simulink model "Marine_LocoMotive_UAV"  (R2018a)
settings: Solver=ode4  StartTime=0.0  StopTime=80  FixedStep=T  RelTol=1e-3
values from neighbouring files (symbols this model uses):
  a_11 = 0.05*m_b    (= 0.625)    [Marine_LocoMotive_UAV.m]
  a_33 = m_b    (= 12.5)    [Marine_LocoMotive_UAV.m]
  A_w = 1*1.5/2    (= 0.75)    [Marine_LocoMotive_UAV.m]
  A_w2 = 1*0.27/2    (= 0.135)    [Marine_LocoMotive_UAV.m]
  Ac = 0.0331    [Marine_LocoMotive_UAV.m]
  alpha_bar = pi/4    (= 0.785398163397)    [Marine_LocoMotive_UAV.m]
  Am = sysd.denominator{1}    [Marine_LocoMotive_UAV.m]
  Am1_LPF = sysd.denominator{1}    [Marine_LocoMotive_UAV.m]
  Am2_LPF = sysd.denominator{1}    [Marine_LocoMotive_UAV.m]
  Am_asw_LPF = sysd.denominator{1}    [Marine_LocoMotive_UAV.m]
  Am_coup_LPF = sysd.denominator{1}    [Marine_LocoMotive_UAV.m]
  Am_rdeL_LPF = sysd.denominator{1}    [Marine_LocoMotive_UAV.m]
  Am_reL_LPF = sysd.denominator{1}    [Marine_LocoMotive_UAV.m]
  Am_rref20_LPF = sysd.denominator{1}    [Marine_LocoMotive_UAV.m]
  Am_rref_LPF = sysd.denominator{1}    [Marine_LocoMotive_UAV.m]
  AmAlpha_LPF = sysd.denominator{1}    [Marine_LocoMotive_UAV.m]
  Amp_sf = 3    [Marine_LocoMotive_UAV.m]
  AmV_LPF = sysd.denominator{1}    [Marine_LocoMotive_UAV.m]
  AmZ_LPF = sysd.denominator{1}    [Marine_LocoMotive_UAV.m]
  b_11 = 0    [Marine_LocoMotive_UAV.m]
  b_33 = 2*m_b*omega_h    (= 27.5578302946)    [Marine_LocoMotive_UAV.m]
  Bm = sysd.numerator{1}    [Marine_LocoMotive_UAV.m]
  Bm1_LPF = sysd.numerator{1}    [Marine_LocoMotive_UAV.m]
  Bm2_LPF = sysd.numerator{1}    [Marine_LocoMotive_UAV.m]
  Bm_asw_LPF = sysd.numerator{1}    [Marine_LocoMotive_UAV.m]
  Bm_coup_LPF = sysd.numerator{1}    [Marine_LocoMotive_UAV.m]
  Bm_rdeL_LPF = sysd.numerator{1}    [Marine_LocoMotive_UAV.m]
  Bm_reL_LPF = sysd.numerator{1}    [Marine_LocoMotive_UAV.m]
  Bm_rref20_LPF = sysd.numerator{1}    [Marine_LocoMotive_UAV.m]
  Bm_rref_LPF = sysd.numerator{1}    [Marine_LocoMotive_UAV.m]
  BmAlpha_LPF = sysd.numerator{1}    [Marine_LocoMotive_UAV.m]
  BmV_LPF = sysd.numerator{1}    [Marine_LocoMotive_UAV.m]
  BmZ_LPF = sysd.numerator{1}    [Marine_LocoMotive_UAV.m]
  C_S = [5;9]*10^-3    [Marine_LocoMotive_UAV.m]
  Cd_u = 0.2    [Marine_LocoMotive_UAV.m]
  D_x = b_11 + D_s(1)    [Marine_LocoMotive_UAV.m]
  D_z = b_33 + D_s(2)    [Marine_LocoMotive_UAV.m]
  dc_M_p = 6.7    [Marine_LocoMotive_UAV.m]
  Delta_h = (A_im/A_b-0.5)*h_b    (= -0.0625)    [Marine_LocoMotive_UAV.m]
  eps_V = 0.1    [Marine_LocoMotive_UAV.m]
  epsilon_1 = 5    [Marine_LocoMotive_UAV.m]
  epsilon_e_u1 = 0.05    [Marine_LocoMotive_UAV.m]
  epsilon_w = 0    [Marine_LocoMotive_UAV.m]
  epsilon_w2 = pi    (= 3.14159265359)    [Marine_LocoMotive_UAV.m]
  g = 9.81    [Marine_LocoMotive_UAV.m]
  gamma_d_p = (2*0.3/0.03*2*0.2*12/4)/10    (= 2.4)    [Marine_LocoMotive_UAV.m]
  H = 10    [Marine_LocoMotive_UAV.m]
  h_b = 0.25    [Marine_LocoMotive_UAV.m]
  J_b = m_b*h_b*l_b/12    (= 0.208333333333)    [Marine_LocoMotive_UAV.m]
  J_u = 0.03    [Marine_LocoMotive_UAV.m]
  K = 40    [Marine_LocoMotive_UAV.m]
  k3 = 24    [Marine_LocoMotive_UAV.m]
  k4 = 0.8    [Marine_LocoMotive_UAV.m]
  k_w = omega_w^2/g    (= 0.123862835563)    [Marine_LocoMotive_UAV.m]
  k_w2 = omega_w2^2/g    (= 0.447144836384)    [Marine_LocoMotive_UAV.m]
  kd_a = 5.6    [Marine_LocoMotive_UAV.m]
  kd_r = 19.5    [Marine_LocoMotive_UAV.m]
  kd_t = 10    [Marine_LocoMotive_UAV.m]
  kd_x = 5    [Marine_LocoMotive_UAV.m]
  kd_z = 2    [Marine_LocoMotive_UAV.m]
  ki_a = 1.6    [Marine_LocoMotive_UAV.m]
  ki_r = 9    [Marine_LocoMotive_UAV.m]
  ki_T = 12    [Marine_LocoMotive_UAV.m]
  ki_x = 1.2    [Marine_LocoMotive_UAV.m]
  ki_z = 1    [Marine_LocoMotive_UAV.m]
  kp_a = 9.6    [Marine_LocoMotive_UAV.m]
  kp_r = 45    [Marine_LocoMotive_UAV.m]
  kp_t = 20    [Marine_LocoMotive_UAV.m]
  kp_T = 25    [Marine_LocoMotive_UAV.m]
  kp_x = 7    [Marine_LocoMotive_UAV.m]
  kp_z = 3    [Marine_LocoMotive_UAV.m]
  L = 0.2    [Marine_LocoMotive_UAV.m]
  l_b = 0.8    [Marine_LocoMotive_UAV.m]
  Lc_0 = 7    [Marine_LocoMotive_UAV.m]
  LIMIT_CMD_PITCH = 45*pi/180    (= 0.785398163397)    [Marine_LocoMotive_UAV.m]
  LIMIT_uCMD_HEIGHT = 3.5*K    (= 140)    [Marine_LocoMotive_UAV.m]
  m_b = rho_w*Vol_b/4    (= 12.5)    [Marine_LocoMotive_UAV.m]
  m_u = 1.8    [Marine_LocoMotive_UAV.m]
  min_sf = 5    [Marine_LocoMotive_UAV.m]
  nu_w = 1.787*10^-6    (= 1.787e-06)    [Marine_LocoMotive_UAV.m]
  omega_w = 2*pi/T_w    (= 1.10231321179)    [Marine_LocoMotive_UAV.m]
  omega_w2 = 2*pi/T_w2    (= 2.09439510239)    [Marine_LocoMotive_UAV.m]
  r_0 = sqrt( (X0_b(1) - X0_u(1))^2 +(X0_b(2) - X0_u(2))^2 )    [Marine_LocoMotive_UAV.m]
  r_bar = Lc_0-0.3    (= 6.7)    [Marine_LocoMotive_UAV.m]
  r_min = (zu_bar-H)-0.2    [Marine_LocoMotive_UAV.m]
  rho_a = 1.225    [Marine_LocoMotive_UAV.m]
  rho_w = 1000    [Marine_LocoMotive_UAV.m]
  T = 1/500    (= 0.002)    [Marine_LocoMotive_UAV.m]
  T_init = 10    [Marine_LocoMotive_UAV.m]
  Theta0 = 0*atan2(V_bar*D_x*cos(alpha_bar_0),V_bar*D_x*sin(alpha_bar_0)+m_u*g*cos(alpha_bar_0))    [Marine_LocoMotive_UAV.m]
  u_s = w_dir*A_w^2*omega_w*k_w*exp(2*k_w*(-Delta_h/2))    [Marine_LocoMotive_UAV.m]
  u_s2 = w_dir2*A_w2^2*omega_w2*k_w2*exp(2*k_w2*(-Delta_h/2))    [Marine_LocoMotive_UAV.m]
  u_t = -1*0.5*1    (= -0.5)    [Marine_LocoMotive_UAV.m]
  u_w = 0*0.2    (= 0)    [Marine_LocoMotive_UAV.m]
  V0_b = [u_t+u_w+u_s+v_x_w, v_z_w]    [Marine_LocoMotive_UAV.m]
  V0_u = [0 0]    [Marine_LocoMotive_UAV.m]
  V_bar = 4    [Marine_LocoMotive_UAV.m]
  Vol_b = A_b*l_b    (= 0.05)    [Marine_LocoMotive_UAV.m]
  w_dir = 1    [Marine_LocoMotive_UAV.m]
  w_dir2 = 1    [Marine_LocoMotive_UAV.m]
  X0_b = [0,H-Delta_h]    [Marine_LocoMotive_UAV.m]
  X0_u = X0_b + [3 3]    [Marine_LocoMotive_UAV.m]
  zu_bar = X0_b(2) + Lc_0*sin(alpha_bar_0)    [Marine_LocoMotive_UAV.m]
undefined symbols (not defined in the file or in its folder): Am_HPF, Am_LPF, Am_LPF2, an1, an1_v, an2, an3, Bm_HPF, Bm_LPF, Bm_LPF2, bn1, bn1_v, bn2, bn3, DiscIntNeverNeededParam, F, Light, magnitude, MIL, OMEGA_FILTER_OUTER, R_b, Tc, Tg, Tn, Ts, Tsc, Tz, X_GPS_offset
libraries: simulink x50, simulink_extras x9, aerolibwind2 x2
(part 6 of 6)

== system Marine_LocoMotive_UAV/UAV controller/u_r_V_Lyapunov buoy velocity/Smooth channel switching1/C1 transition ==
  C1 : Inport
  switch : Inport  Port=2
  C2_0 : Inport  Port=3
  Compare To Constant : simulink/Logic and Bit Operations/Compare To Constant  relop=<  const=0.01  OutDataTypeStr=boolean
  Constant : Constant
  Constant1 : Constant  Value=0.01
  Delay1 : Delay  DelayLength=1
  IC : InitialCondition  Value=0
  Logical Operator : Logic  Operator=NOT  AllPortsSameDT=off  OutDataTypeStr=boolean
  Product : Product
  Subsystem : Subsystem
  Sum : Sum  Inputs=-+|
  Sum1 : Sum  Inputs=++|
  Sum3 : Sum  Inputs=|++
  Switch1 : Switch  Criteria=u2 > Threshold  Threshold=0.5
  Switch2 : Switch  Criteria=u2 > Threshold  Threshold=0.5
  latch : Subsystem  TreatAsAtomicUnit=on
  latch error ON : Scope
  record C2_0 : Subsystem  TreatAsAtomicUnit=on
  smooth transition to C1 : Subsystem  TreatAsAtomicUnit=on
  trigger and reset latch : Subsystem
  C1_trans : Outport
  wires:
  trigger and reset latch/1(Out1) -> latch/Trigger
  Logical Operator/1 -> Product/2
  IC/1 -> latch/1(In1), trigger and reset latch/2(In2)
  switch/1 -> smooth transition to C1/Enable, Subsystem/Enable, trigger and reset latch/1(In1), record C2_0/Trigger, Delay1/1, Logical Operator/1, Switch2/2
  Sum/1 -> smooth transition to C1/1(In1)
  Delay1/1 -> smooth transition to C1/2(reset)
  Compare To Constant/1 -> IC/1
  Subsystem/1(Out1) -> Sum3/1
  Sum3/1 -> Compare To Constant/1
  Product/1 -> Sum3/2  "do not latch C1 is off"
  Constant1/1 -> Product/1
  Constant/1 -> Switch2/3
  Switch2/1 -> latch error ON/1, Switch1/2
  latch/1(Out1) -> Switch2/1
  Switch1/1 -> C1_trans/1  "out"
  C1/1 -> Sum/2, Switch1/1, Subsystem/2(C1)  "C1"
  record C2_0/1(Out1) -> Sum1/1, Sum/1  "C2_0"
  smooth transition to C1/1(Out1) -> Sum1/2
  C2_0/1 -> record C2_0/1(In1)
  Sum1/1 -> Switch1/3, Subsystem/1(addition with C2_0)  "addition with C2_0"

== system Marine_LocoMotive_UAV/UAV controller/u_r_V_Lyapunov buoy velocity/Smooth channel switching1/C2 transition ==
  C2 : Inport
  switch : Inport  Port=2
  C1_0 : Inport  Port=3
  Compare To Constant : simulink/Logic and Bit Operations/Compare To Constant  relop=<  const=0.01  OutDataTypeStr=boolean
  Constant : Constant
  Constant1 : Constant  Value=0.01
  Delay1 : Delay  DelayLength=1
  Logical Operator : Logic  Operator=NOT  AllPortsSameDT=off  OutDataTypeStr=boolean
  Product : Product
  Subsystem : Subsystem
  Sum : Sum  Inputs=-+|
  Sum1 : Sum  Inputs=++|
  Sum3 : Sum  Inputs=|++
  Switch1 : Switch  Criteria=u2 > Threshold  Threshold=0.5
  Switch2 : Switch  Criteria=u2 > Threshold  Threshold=0.5
  latch : Subsystem  TreatAsAtomicUnit=on
  latch error ON : Scope
  record C1_0 : Subsystem  TreatAsAtomicUnit=on
  smooth transition to C1 : Subsystem  TreatAsAtomicUnit=on
  trigger and reset latch : Subsystem
  C2_trans : Outport
  wires:
  trigger and reset latch/1(Out1) -> latch/Trigger
  Compare To Constant/1 -> latch/1(In1), trigger and reset latch/2(In2)
  Subsystem/1(Out1) -> Sum3/1
  Delay1/1 -> smooth transition to C1/2(reset)
  Logical Operator/1 -> Product/2
  Sum3/1 -> Compare To Constant/1
  Constant1/1 -> Product/1
  Product/1 -> Sum3/2
  latch/1(Out1) -> Switch2/1
  Constant/1 -> Switch2/3
  Sum1/1 -> Switch1/3, Subsystem/1(addition with C1_0)  "addition with C1_0"
  C1_0/1 -> record C1_0/1(In1)
  smooth transition to C1/1(Out1) -> Sum1/2
  record C1_0/1(Out1) -> Sum/1, Sum1/1  "C1_0"
  switch/1 -> record C1_0/Trigger, trigger and reset latch/1(trigger), Subsystem/Enable, smooth transition to C1/Enable, Delay1/1, Logical Operator/1, Switch2/2  "trigger"
  Switch2/1 -> latch error ON/1, Switch1/2
  C2/1 -> Switch1/1, Subsystem/2(C2), Sum/2  "C2"
  Switch1/1 -> C2_trans/1  "out"
  Sum/1 -> smooth transition to C1/1(In1)

== system Marine_LocoMotive_UAV/Quadrotor+buoy/3-DOF equations of motion Earth frame/D_123/Water Daming/rotation matrix R body to earth ==
  angle (rad) : Inport
  Gain : Gain  Gain=-1
  Signal Specification1 : SignalSpecification  Dimensions=2
  Signal Specification2 : SignalSpecification  Dimensions=2
  Trigonometric Function1 : Trigonometry  Operator=sincos
  Vector Concatenate1 : Concatenate  Mode=Multidimensional array  ConcatenateDimension=2
  Vector Concatenate2 : Concatenate
  Vector Concatenate3 : Concatenate
  R : Outport
  wires:
  Gain/1 -> Vector Concatenate3/1
  Trigonometric Function1/1 -> Gain/1, Vector Concatenate2/2
  Trigonometric Function1/2 -> Vector Concatenate2/1, Vector Concatenate3/2
  angle (rad)/1 -> Trigonometric Function1/1
  Vector Concatenate3/1 -> Signal Specification2/1
  Vector Concatenate2/1 -> Signal Specification1/1
  Vector Concatenate1/1 -> R/1
  Signal Specification1/1 -> Vector Concatenate1/1
  Signal Specification2/1 -> Vector Concatenate1/2

== system Marine_LocoMotive_UAV/Quadrotor+buoy/3-DOF equations of motion Earth frame/Quadrotor Dynamics Outer-Loop/quadrotor position from relative buoy-UAV position/rotation matrix R  ==
  angle (rad) : Inport
  Gain2 : Gain  Gain=-1
  Gain3 : Gain  Gain=-1
  Signal Specification1 : SignalSpecification  Dimensions=2
  Signal Specification2 : SignalSpecification  Dimensions=2
  Trigonometric Function1 : Trigonometry  Operator=sincos
  Vector Concatenate1 : Concatenate  Mode=Multidimensional array  ConcatenateDimension=2
  Vector Concatenate2 : Concatenate
  Vector Concatenate3 : Concatenate
  R : Outport
  wires:
  Signal Specification2/1 -> Vector Concatenate1/2
  Signal Specification1/1 -> Vector Concatenate1/1
  Vector Concatenate1/1 -> R/1
  Vector Concatenate2/1 -> Signal Specification1/1
  Vector Concatenate3/1 -> Signal Specification2/1
  angle (rad)/1 -> Trigonometric Function1/1
  Trigonometric Function1/1 -> Gain3/1
  Trigonometric Function1/2 -> Vector Concatenate3/2, Gain2/1
  Gain3/1 -> Vector Concatenate2/2, Vector Concatenate3/1
  Gain2/1 -> Vector Concatenate2/1

== system Marine_LocoMotive_UAV/Quadrotor+buoy/3-DOF equations of motion Earth frame/azimuthal dynamics/Coupled System's azimuthal dynamics/azimuth angle dynamics in the coupled system ==
  alpha_ddot : Inport
  alpha init : Inport  Port=2
  alpha dot init : Inport  Port=3
  reset : Inport  Port=4
  Enable : EnablePort
  " alpha" : Scope
  " alpha dot" : Scope
  " alpha dot init" : Scope
  " alpha init" : Scope
  alpha : DiscreteIntegrator  IntegratorMethod=Integration: Backward Euler  ExternalReset=level  InitialConditionSource=external  InitialCondition=alpha_0  SampleTime=-1  ICPrevOutput=DiscIntNeverNeededParam  ICPrevScaledInput=DiscIntNeverNeededParam
  dot(alpha) : DiscreteIntegrator  IntegratorMethod=Integration: Backward Euler  ExternalReset=level  InitialConditionSource=external  SampleTime=-1  ICPrevOutput=DiscIntNeverNeededParam  ICPrevScaledInput=DiscIntNeverNeededParam
  "reset " : Scope
  "alpha " : Outport
  alpha dot : Outport  Port=2
  wires:
  dot(alpha)/1 -> alpha/1, " alpha dot"/1, alpha dot/1
  alpha_ddot/1 -> dot(alpha)/1
  alpha/1 -> "alpha "/1, " alpha"/1
  alpha dot init/1 -> " alpha dot init"/1, dot(alpha)/3
  alpha init/1 -> " alpha init"/1, alpha/3
  reset/1 -> "reset "/1, alpha/2, dot(alpha)/2

== system Marine_LocoMotive_UAV/Quadrotor+buoy/3-DOF equations of motion Earth frame/azimuthal dynamics/Coupled System's azimuthal dynamics/get initial azimuth angle for the coupled dynamics ==
  alpha decoupled : Inport
  alpha dot decoupled : Inport  Port=2
  Trigger : TriggerPort  VariantControl=Variant
  alpha init : Outport
  alpha dot init : Outport  Port=2
  wires:
  alpha decoupled/1 -> alpha init/1
  alpha dot decoupled/1 -> alpha dot init/1

== system Marine_LocoMotive_UAV/Quadrotor+buoy/3-DOF equations of motion Earth frame/azimuthal dynamics/Decoupled System's azimuthal dynamics/magnitude ==
  dX : Inport
  Math Function2 : Math  Operator=square  SaturateOnIntegerOverflow=on
  Sqrt : Sqrt  SaturateOnIntegerOverflow=on
  Sum of Elements : Sum  Inputs=+
  r : Outport
  wires:
  Math Function2/1 -> Sum of Elements/1
  Sum of Elements/1 -> Sqrt/1
  dX/1 -> Math Function2/1
  Sqrt/1 -> r/1

== system Marine_LocoMotive_UAV/Quadrotor+buoy/3-DOF equations of motion Earth frame/azimuthal dynamics/Decoupled System's azimuthal dynamics/rotation matrix R  ==
  angle (rad) : Inport
  Gain : Gain  Gain=-1
  Signal Specification1 : SignalSpecification  Dimensions=2
  Signal Specification2 : SignalSpecification  Dimensions=2
  Trigonometric Function1 : Trigonometry  Operator=sincos
  Vector Concatenate1 : Concatenate  Mode=Multidimensional array  ConcatenateDimension=2
  Vector Concatenate2 : Concatenate
  Vector Concatenate3 : Concatenate
  R : Outport
  wires:
  Signal Specification2/1 -> Vector Concatenate1/2
  Signal Specification1/1 -> Vector Concatenate1/1
  Vector Concatenate1/1 -> R/1
  Vector Concatenate2/1 -> Signal Specification1/1
  Vector Concatenate3/1 -> Signal Specification2/1
  angle (rad)/1 -> Trigonometric Function1/1
  Trigonometric Function1/2 -> Vector Concatenate3/2, Vector Concatenate2/1
  Trigonometric Function1/1 -> Vector Concatenate2/2, Gain/1
  Gain/1 -> Vector Concatenate3/1

== system Marine_LocoMotive_UAV/Quadrotor+buoy/3-DOF equations of motion Earth frame/azimuthal dynamics/Decoupled System's azimuthal dynamics/rotation matrix R 1 ==
  angle (rad) : Inport
  Gain : Gain  Gain=-1
  Signal Specification1 : SignalSpecification  Dimensions=2
  Signal Specification2 : SignalSpecification  Dimensions=2
  Trigonometric Function1 : Trigonometry  Operator=sincos
  Vector Concatenate1 : Concatenate  Mode=Multidimensional array  ConcatenateDimension=2
  Vector Concatenate2 : Concatenate
  Vector Concatenate3 : Concatenate
  R : Outport
  wires:
  Gain/1 -> Vector Concatenate3/1
  Trigonometric Function1/1 -> Gain/1, Vector Concatenate2/2
  Trigonometric Function1/2 -> Vector Concatenate2/1, Vector Concatenate3/2
  angle (rad)/1 -> Trigonometric Function1/1
  Vector Concatenate3/1 -> Signal Specification2/1
  Vector Concatenate2/1 -> Signal Specification1/1
  Vector Concatenate1/1 -> R/1
  Signal Specification1/1 -> Vector Concatenate1/1
  Signal Specification2/1 -> Vector Concatenate1/2

== system Marine_LocoMotive_UAV/Sensors and Filters/Sensors/ Sonar (10Hz) (true elevation instead real sonar signal)/Sampler/Triggered Subsystem ==
  In1 : Inport
  Trigger : TriggerPort  VariantControl=(inherit)
  Out1 : Outport
  wires:
  In1/1 -> Out1/1

== system Marine_LocoMotive_UAV/UAV controller/switch controllers/Smooth channel switching/C1 transition/Subsystem ==
  addition with C2_0 : Inport
  C1 : Inport  Port=2
  Enable : EnablePort
  Abs : Abs
  Sum2 : Sum  Inputs=-+|
  Out1 : Outport
  wires:
  addition with C2_0/1 -> Sum2/1
  C1/1 -> Sum2/2
  Sum2/1 -> Abs/1  "calculate the error"
  Abs/1 -> Out1/1

== system Marine_LocoMotive_UAV/UAV controller/switch controllers/Smooth channel switching/C1 transition/latch ==
  In1 : Inport
  Trigger : TriggerPort  VariantControl=Variant
  Out1 : Outport
  wires:
  In1/1 -> Out1/1

== system Marine_LocoMotive_UAV/UAV controller/switch controllers/Smooth channel switching/C1 transition/record C2_0 ==
  In1 : Inport
  Trigger : TriggerPort  TriggerType=either  VariantControl=Variant
  Out1 : Outport
  wires:
  In1/1 -> Out1/1

== system Marine_LocoMotive_UAV/UAV controller/switch controllers/Smooth channel switching/C1 transition/smooth transition to C1 ==
  In1 : Inport
  reset : Inport  Port=2
  Enable : EnablePort
  Discrete Transfer Fcn1 : DiscreteTransferFcn  Numerator=Bm_coup_LPF  Denominator=Am_coup_LPF  ExternalReset=Either
      settings: InputPortMap=u0,r7
  Out1 : Outport
  wires:
  Discrete Transfer Fcn1/1 -> Out1/1
  In1/1 -> Discrete Transfer Fcn1/1
  reset/1 -> Discrete Transfer Fcn1/2

== system Marine_LocoMotive_UAV/UAV controller/switch controllers/Smooth channel switching/C1 transition/trigger and reset latch ==
  In1 : Inport
  In2 : Inport  Port=2
  Abs : Abs
  Add : Sum
  Data Type Conversion : DataTypeConversion
  Data Type Conversion1 : DataTypeConversion
  Discrete Derivative1 : simulink/Discrete/Discrete Derivative  gainval=1.0  ICPrevScaledInput=0.0  OutMin=[]  OutMax=[]  OutDataType=fixdt(1, 16)  OutScaling=2^-10  DoSatur=off
  IC1 : InitialCondition  Value=0
  Saturation : Saturate  UpperLimit=1  LowerLimit=0
  Out1 : Outport
  wires:
  IC1/1 -> Saturation/1
  Discrete Derivative1/1 -> Abs/1
  In2/1 -> Data Type Conversion/1
  Abs/1 -> IC1/1
  Add/1 -> Out1/1
  Data Type Conversion1/1 -> Discrete Derivative1/1
  Saturation/1 -> Add/1
  Data Type Conversion/1 -> Add/2
  In1/1 -> Data Type Conversion1/1

== system Marine_LocoMotive_UAV/UAV controller/switch controllers/Smooth channel switching/C2 transition/Subsystem ==
  addition with C1_0 : Inport
  C2 : Inport  Port=2
  Enable : EnablePort
  Abs : Abs
  Sum2 : Sum  Inputs=-+|
  Out1 : Outport
  wires:
  addition with C1_0/1 -> Sum2/1
  Sum2/1 -> Abs/1  "calculate the error"
  Abs/1 -> Out1/1
  C2/1 -> Sum2/2

== system Marine_LocoMotive_UAV/UAV controller/switch controllers/Smooth channel switching/C2 transition/latch ==
  In1 : Inport
  Trigger : TriggerPort  VariantControl=Variant
  Out1 : Outport
  wires:
  In1/1 -> Out1/1

== system Marine_LocoMotive_UAV/UAV controller/switch controllers/Smooth channel switching/C2 transition/record C1_0 ==
  In1 : Inport
  Trigger : TriggerPort  VariantControl=Variant
  Out1 : Outport
  wires:
  In1/1 -> Out1/1

== system Marine_LocoMotive_UAV/UAV controller/switch controllers/Smooth channel switching/C2 transition/smooth transition to C1 ==
  In1 : Inport
  reset : Inport  Port=2
  Enable : EnablePort
  Discrete Transfer Fcn1 : DiscreteTransferFcn  Numerator=Bm_coup_LPF  Denominator=Am_coup_LPF  ExternalReset=Either
      settings: InputPortMap=u0,r7
  Out1 : Outport
  wires:
  Discrete Transfer Fcn1/1 -> Out1/1
  In1/1 -> Discrete Transfer Fcn1/1
  reset/1 -> Discrete Transfer Fcn1/2

== system Marine_LocoMotive_UAV/UAV controller/switch controllers/Smooth channel switching/C2 transition/trigger and reset latch ==
  trigger : Inport
  In2 : Inport  Port=2
  Abs : Abs
  Add : Sum
  Data Type Conversion : DataTypeConversion
  Data Type Conversion1 : DataTypeConversion
  Discrete Derivative1 : simulink/Discrete/Discrete Derivative  gainval=1.0  ICPrevScaledInput=0.0  OutMin=[]  OutMax=[]  OutDataType=fixdt(1, 16)  OutScaling=2^-10  DoSatur=off
  IC1 : InitialCondition  Value=0
  Saturation : Saturate  UpperLimit=1  LowerLimit=0
  Out1 : Outport
  wires:
  trigger/1 -> Data Type Conversion1/1
  Add/1 -> Out1/1
  Abs/1 -> IC1/1
  Data Type Conversion/1 -> Add/2
  In2/1 -> Data Type Conversion/1
  Saturation/1 -> Add/1
  Discrete Derivative1/1 -> Abs/1
  Data Type Conversion1/1 -> Discrete Derivative1/1
  IC1/1 -> Saturation/1

== system Marine_LocoMotive_UAV/UAV controller/u_r_V_Lyapunov buoy velocity/Smooth channel switching1/C1 transition/Subsystem ==
  addition with C2_0 : Inport
  C1 : Inport  Port=2
  Enable : EnablePort
  Abs : Abs
  Sum2 : Sum  Inputs=-+|
  Out1 : Outport
  wires:
  Abs/1 -> Out1/1
  Sum2/1 -> Abs/1  "calculate the error"
  C1/1 -> Sum2/2
  addition with C2_0/1 -> Sum2/1

== system Marine_LocoMotive_UAV/UAV controller/u_r_V_Lyapunov buoy velocity/Smooth channel switching1/C1 transition/latch ==
  In1 : Inport
  Trigger : TriggerPort  VariantControl=Variant
  Out1 : Outport
  wires:
  In1/1 -> Out1/1

== system Marine_LocoMotive_UAV/UAV controller/u_r_V_Lyapunov buoy velocity/Smooth channel switching1/C1 transition/record C2_0 ==
  In1 : Inport
  Trigger : TriggerPort  TriggerType=either  VariantControl=Variant
  Out1 : Outport
  wires:
  In1/1 -> Out1/1

== system Marine_LocoMotive_UAV/UAV controller/u_r_V_Lyapunov buoy velocity/Smooth channel switching1/C1 transition/smooth transition to C1 ==
  In1 : Inport
  reset : Inport  Port=2
  Enable : EnablePort
  Discrete Transfer Fcn1 : DiscreteTransferFcn  Numerator=Bm_coup_LPF  Denominator=Am_coup_LPF  ExternalReset=Either
      settings: InputPortMap=u0,r7
  Out1 : Outport
  wires:
  reset/1 -> Discrete Transfer Fcn1/2
  In1/1 -> Discrete Transfer Fcn1/1
  Discrete Transfer Fcn1/1 -> Out1/1

== system Marine_LocoMotive_UAV/UAV controller/u_r_V_Lyapunov buoy velocity/Smooth channel switching1/C1 transition/trigger and reset latch ==
  In1 : Inport
  In2 : Inport  Port=2
  Abs : Abs
  Add : Sum
  Data Type Conversion : DataTypeConversion
  Data Type Conversion1 : DataTypeConversion
  Discrete Derivative1 : simulink/Discrete/Discrete Derivative  gainval=1.0  ICPrevScaledInput=0.0  OutMin=[]  OutMax=[]  OutDataType=fixdt(1, 16)  OutScaling=2^-10  DoSatur=off
  IC1 : InitialCondition  Value=0
  Saturation : Saturate  UpperLimit=1  LowerLimit=0
  Out1 : Outport
  wires:
  In1/1 -> Data Type Conversion1/1
  Data Type Conversion/1 -> Add/2
  Saturation/1 -> Add/1
  Data Type Conversion1/1 -> Discrete Derivative1/1
  Add/1 -> Out1/1
  Abs/1 -> IC1/1
  In2/1 -> Data Type Conversion/1
  Discrete Derivative1/1 -> Abs/1
  IC1/1 -> Saturation/1

== system Marine_LocoMotive_UAV/UAV controller/u_r_V_Lyapunov buoy velocity/Smooth channel switching1/C2 transition/Subsystem ==
  addition with C1_0 : Inport
  C2 : Inport  Port=2
  Enable : EnablePort
  Abs : Abs
  Sum2 : Sum  Inputs=-+|
  Out1 : Outport
  wires:
  C2/1 -> Sum2/2
  Abs/1 -> Out1/1
  Sum2/1 -> Abs/1  "calculate the error"
  addition with C1_0/1 -> Sum2/1

== system Marine_LocoMotive_UAV/UAV controller/u_r_V_Lyapunov buoy velocity/Smooth channel switching1/C2 transition/latch ==
  In1 : Inport
  Trigger : TriggerPort  VariantControl=Variant
  Out1 : Outport
  wires:
  In1/1 -> Out1/1

== system Marine_LocoMotive_UAV/UAV controller/u_r_V_Lyapunov buoy velocity/Smooth channel switching1/C2 transition/record C1_0 ==
  In1 : Inport
  Trigger : TriggerPort  VariantControl=Variant
  Out1 : Outport
  wires:
  In1/1 -> Out1/1

== system Marine_LocoMotive_UAV/UAV controller/u_r_V_Lyapunov buoy velocity/Smooth channel switching1/C2 transition/smooth transition to C1 ==
  In1 : Inport
  reset : Inport  Port=2
  Enable : EnablePort
  Discrete Transfer Fcn1 : DiscreteTransferFcn  Numerator=Bm_coup_LPF  Denominator=Am_coup_LPF  ExternalReset=Either
      settings: InputPortMap=u0,r7
  Out1 : Outport
  wires:
  reset/1 -> Discrete Transfer Fcn1/2
  In1/1 -> Discrete Transfer Fcn1/1
  Discrete Transfer Fcn1/1 -> Out1/1

== system Marine_LocoMotive_UAV/UAV controller/u_r_V_Lyapunov buoy velocity/Smooth channel switching1/C2 transition/trigger and reset latch ==
  trigger : Inport
  In2 : Inport  Port=2
  Abs : Abs
  Add : Sum
  Data Type Conversion : DataTypeConversion
  Data Type Conversion1 : DataTypeConversion
  Discrete Derivative1 : simulink/Discrete/Discrete Derivative  gainval=1.0  ICPrevScaledInput=0.0  OutMin=[]  OutMax=[]  OutDataType=fixdt(1, 16)  OutScaling=2^-10  DoSatur=off
  IC1 : InitialCondition  Value=0
  Saturation : Saturate  UpperLimit=1  LowerLimit=0
  Out1 : Outport
  wires:
  IC1/1 -> Saturation/1
  Data Type Conversion1/1 -> Discrete Derivative1/1
  Discrete Derivative1/1 -> Abs/1
  Saturation/1 -> Add/1
  In2/1 -> Data Type Conversion/1
  Data Type Conversion/1 -> Add/2
  Abs/1 -> IC1/1
  Add/1 -> Out1/1
  trigger/1 -> Data Type Conversion1/1

== matlab function Marine_LocoMotive_UAV/Quadrotor+buoy/3-DOF equations of motion Earth frame/Coupling state/MATLAB Function ==
  data: pos_T input; is_coupled output; re_couple input; coupled input; c output
function [is_coupled,c] = fcn(pos_T, re_couple, coupled)

% persistent coupled
% if isempty(coupled) 
%     coupled = 1;
% end

if and(pos_T == 1 , coupled == 1)
    coupled = 1;
    c = 1; 
    
elseif and(pos_T == 0 , coupled == 1)
    coupled = 0;
    c = 2;
elseif and(coupled == 0 , re_couple == 0)
    coupled = 0;
    c = 3;
elseif and(coupled == 0 , re_couple == 1)
    coupled = 1;
    c = 4;
elseif and(pos_T == 0 , coupled == 0)
    coupled = 0;
    c = 5;
else
    coupled = 1;
    c = 6;
end
    
is_coupled = coupled;

== matlab function Marine_LocoMotive_UAV/Sensors and Filters/Data processing/Estimate Attitude/Kalman Filter - Pitch ==
  settings: updateMethod=DISCRETE  sampleTime=T
  data: angle output; acc_angle input; gyro_rate input; opti_angle input; dt input
function angle   = fcn(acc_angle,gyro_rate,opti_angle,dt)
%#eml
    % a bias in the accelerometer will result in a bias in the filter
    % estimate
    Q_angle = 0.001;
    Q_gyro   = 0.001; %0.01;  %0.003
    R_angle  =  0.01;  %0.03

    
    persistent P_00;
    persistent P_01;
    persistent P_10;
    persistent P_11;
    persistent x_angle;
    persistent x_bias;
        
    if isempty(P_00)
        P_00 = 1.5*10^-4;
    end
    
    if isempty(P_01)
        P_01 = -1.4*10^-4;
    end
    if isempty(P_10)
        P_10 = -1.4*10^-4;
    end
    if isempty(P_11)
        P_11 = 11.4*10^-4;
    end
     if isempty(x_bias)
        x_bias = 0;
     end
     if isempty(x_angle)
        x_angle = 0;
     end
    
    
    % Calculate the new output
    x_angle = x_angle + dt * (gyro_rate - x_bias);%
    P_00 = P_00 -  dt * (P_10 + P_01) + Q_angle * dt;
    P_01 = P_01  - dt * P_11;
    P_10 = P_10  - dt * P_11;
    P_11 = P_11  + Q_gyro * dt;

    % Assuming H = [0.98 (effect of gyro) 0.02 (effect of acc)]
    %e = (0.97*x_angle + 0.03*acc_angle) - x_angle;
    e = (0.9*x_angle + 0.001*acc_angle + 0.099*opti_angle) - x_angle;
    S = P_00 + R_angle;
    K_0 = P_00 / S;
    K_1 = P_10 / S;

    % Correction
    x_angle = x_angle+  K_0 * e;
    x_bias  = x_bias+  K_1 * e;
    P_00 = P_00 - K_0 * P_00;
    P_01 = P_01 - K_0 * P_01;
    P_10 = P_10 - K_1 * P_00;
    P_11 = P_11 - K_1 * P_01;

    angle = x_angle;
%     P = [P_00 P_01; P_10 P_11];

== matlab function Marine_LocoMotive_UAV/Sensors and Filters/Coupling detection by r/Coupling state/MATLAB Function ==
  data: pos_T input; is_coupled output; re_couple input; coupled input; c output
function [is_coupled,c] = fcn(pos_T, re_couple, coupled)

% persistent coupled
% if isempty(coupled) 
%     coupled = 1;
% end

if and(pos_T == 1 , coupled == 1)
    coupled = 1;
    c = 1; 
    
elseif and(pos_T == 0 , coupled == 1)
    coupled = 0;
    c = 2;
elseif and(coupled == 0 , re_couple == 0)
    coupled = 0;
    c = 3;
elseif and(coupled == 0 , re_couple == 1)
    coupled = 1;
    c = 4;
elseif and(pos_T == 0 , coupled == 0)
    coupled = 0;
    c = 5;
else
    coupled = 1;
    c = 6;
end
    
is_coupled = coupled;

== matlab function Marine_LocoMotive_UAV/Sensors and Filters/Data processing/Estimate Position/Extrapolation - x ==
  settings: updateMethod=DISCRETE
  data: xin input; xout output; xdotin input; dt input; new input; isTracking input; x0 input
function xout = fcn(xin, xdotin, dt, new, isTracking,x0)
%#codegen

%
% Pass through input if "new" data available and OptiTrack is tracking.
% Otherwise, use linear interpolation to estimate the signal value and
% ignore the input data.
%
persistent x;

if( isempty(x) )
    x = x0;
end;

if( new == 1 && isTracking == 1 )
    x = xin;
else
    x = x+dt*xdotin;
end;

xout = x;

== matlab function Marine_LocoMotive_UAV/Refenrence Commands/setpoint velocity controller ==
  settings: updateMethod=DISCRETE
  data: eps input; r input; er_thr input; V_bar_out output; Lc0 input; c output; V0_bar input; V input
function [V_bar_out,c] = fcn(eps,r, er_thr, Lc0, V0_bar, V)%,...
            %c_sm, reset)

persistent V0_old
if isempty(V0_old) 
    V0_old = 0;
end

eps = abs(eps); % make sure that eps is positive.

% Velocity error is low, no output.
if (V0_bar - V <  eps) && (V0_bar - V >=  0)
    V_bar_out = V0_old;
    % return previous V0
    c = 0; 
% Velocity error is high, output the velocity only if the UAV is ready.
elseif (V0_bar - V >=  eps) && (Lc0 - r < er_thr)
    V_bar_out = V0_bar;
    % follow new V0
    c = 1;     
% Velocity error is low, no output.
elseif (V0_bar - V >  -eps) && (V0_bar - V <  0)
    V_bar_out = V0_old;
    % return previous V0
    c = 2; 
% Velocity error is high, output the velocity only if the UAV is ready.
elseif (V0_bar - V <=  -eps) && (Lc0 - r < er_thr)
    V_bar_out = V0_bar;
    % follow new V0
    c = 3;
else  % Velocity error is high, but UAV is not ready
    V_bar_out = V0_old;
    c = 4;
end

% when the new reference velocity is sent to the ouptut,
% set the old reference velocity to the current reference velocty
% to be the zero point when the reference velocty changes again.
if  V_bar_out == V0_bar
    V0_old = V0_bar;
end

== matlab function Marine_LocoMotive_UAV/Sensors and Filters/Data processing/Estimate Position/Extrapolation - z ==
  settings: updateMethod=DISCRETE  sampleTime=T
  data: xin input; xout output; xdotin input; dt input; new input; isTracking input; x0 input
function xout = fcn(xin, xdotin, dt, new, isTracking,x0)
%#codegen

%
% Pass through input if "new" data available and OptiTrack is tracking.
% Otherwise, use linear interpolation to estimate the signal value and
% ignore the input data.
%
persistent x;

if( isempty(x) )
    x = x0;
end

if( new == 1 && isTracking == 1 )
    x = xin;
else
    x = x+dt*xdotin;
end

xout = x;

== matlab function Marine_LocoMotive_UAV/UAV controller/cond1/MATLAB Function ==
  settings: updateMethod=DISCRETE
  data: r input; r_dot input; y output; coupled input; Lc input; dt input; t output
function [y,t]  = fcn(r,r_dot,coupled,Lc,dt)

persistent key
persistent timer

if isempty(key)
    key = 0;
end

if isempty(timer)
    timer = 0;
end

if (r > Lc - 0.1) && (r_dot > 0.25) && (key == 0)
    key = 1;
end

if (r < Lc - 0.12) && (r_dot < -0.1) && (key == 1)
    key = 0;
end

if (key == 1) && (coupled == 1)
    timer = timer + dt;
end

if (timer >= 1) % reset
    key = 0;
    timer = 0;
end

y = key;
t = timer;

== matlab function Marine_LocoMotive_UAV/UAV controller/u_a_Lyapunov/Subsystem1/cond1/MATLAB Function ==
  data: r input; r_dot input; y output; coupled input; Lc input; dt input; t output
function [y,t]  = fcn(r,r_dot,coupled,Lc,dt)

persistent key
persistent timer

if isempty(key)
    key = 0;
end

if isempty(timer)
    timer = 0;
end

if (r > Lc - 0.1) && (r_dot > 0.25) && (key == 0)
    key = 1;
end

if (r < Lc - 0.12) && (r_dot < -0.1) && (key == 1)
    key = 0;
end

if (key == 1) && (coupled == 1)
    timer = timer + dt;
end

if (timer >= 1) % reset
    key = 0;
    timer = 0;
end

y = key;
t = timer;

== matlab function Marine_LocoMotive_UAV/UAV controller/State Machine new ==
  settings: updateMethod=DISCRETE  sampleTime=T
  data: eps input; r input; r_thr input; active output; decelerate output; switch_side output; xdot_b input; V_bar0 input; c output; V_bar input; V_bar_dot input; alpha input; alpha_bar input; x_rel_final input; x_rel input; reset input
function [active,decelerate,switch_side,c] = fcn(eps,r, r_thr, ...
    xdot_b, V_bar0, V_bar, V_bar_dot, alpha, alpha_bar, x_rel_final, x_rel...
    , reset)

persistent state
persistent is_active
persistent decelerating
persistent switching_side

if isempty(is_active) 
    state = 0;
    is_active = 0;
    decelerating = 0;
    switching_side = 0;
end

eps = abs(eps); % make sure that eps is positive.
eps_p1 = 2*eps;
eps_p2 = 2.5*eps;
eps_n1 = 1.5*eps;
eps_n2 = 2*eps;

dx_thr = 0.13;  
% deactivate the velocity controller while reset is on:
if (reset == 1)
    is_active = 0;
    decelerating = 0;
    switching_side = 0;
    % idel state
    state = 0; 
% buoy velocity is low, activate to accelerate:
elseif and( is_active == 0 && decelerating == 0 && switching_side == 0,...
        and( xdot_b <= V_bar0-eps_n1, alpha < pi/2 ) ) 
    is_active = 1;
    % accelerate flag state
    state = 1;     
% % keep activated while pursuing the desired velocity    
% elseif and( is_active == 1 && decelerating == 0 && switching_side == 0 && V_bar_dot >= 0,...
%         and( xdot_b < V_bar+eps_p1, alpha < pi/2 ) ) 
%     is_active = 1;
%     decelerating = 0; 
%     switching_side = 0;
%     % accelerating state
%     c = 2; 
% elseif and( is_active == 1 && decelerating == 0 && switching_side == 0 && V_bar_dot < 0,...,...
%         and( xdot_b < V_bar+eps_n1, alpha < pi/2 ) ) 
%     is_active = 1;
%     decelerating = 0; 
%     switching_side = 0;
%     % accelerating state
%     c = 2.5;     
% deactivate since velocity has gone too high or the system has
% unintentionnally decouple to prevent damage (removed for testing):
elseif and( is_active == 1 && decelerating == 0 && switching_side == 0 && V_bar_dot >= 0,...
        or( (xdot_b >= V_bar+eps_p1), 0 )) % (r < r_thr)
    is_active = 0;
    % acceleration stop state
    state = 2;
elseif and( is_active == 1 && decelerating == 0 && switching_side == 0 && V_bar_dot < 0,...
        or( (xdot_b >= V_bar+eps_n1), (r < r_thr) )) % (r < r_thr)
    is_active = 0;
    % acceleration stop state
    state = 3;    
% % keep deactivated since velocity error has not reached the 
% % upper and lower thresholds:    
% elseif and( is_active==0  && decelerating==0 && switching_side==0 && alpha<pi/2 && V_bar_dot >= 0,...
%         and(xdot_b > V_bar-eps_n1 , xdot_b < V_bar+eps_p2 ) ) 
%     is_active = 0;
%     decelerating = 0; 
%     switching_side = 0;
%     % forward elevation-hold state
%     c = 4;
% elseif and( is_active==0  && decelerating==0 && switching_side==0 && alpha<pi/2 && V_bar_dot < 0,...
%         and(xdot_b > V_bar-eps_n1 , xdot_b < V_bar+0.6*eps_n1 ) ) 
%     is_active = 0;
%     decelerating = 0; 
%     switching_side = 0;
%     % forward elevation-hold state
%     c = 4.5;    
% % prepare to decelerate since velocity is too high:    
% elseif and( is_active == 0  && decelerating == 0 && switching_side == 0 && V_bar_dot >= 0,...
%         and( xdot_b >= V_bar0+eps_p2, alpha < pi/2 ) )  
%     is_active = 0;
%     decelerating = 1; 
%     switching_side = 0;
%     % decelerate flag state
%     c = 5;     
% elseif and( is_active == 0  && decelerating == 0 && switching_side == 0 && V_bar_dot < 0,...
%         and( xdot_b >= V_bar0+0.6*eps_n1, alpha < pi/2 ) )  
%     is_active = 0;
%     decelerating = 1; 
%     switching_side = 0;
%     % decelerate flag state
%     c = 5.5;    
% declare UAV switching side state:    
elseif and( is_active == 0 && decelerating == 0 && switching_side == 0 && V_bar_dot < 0,...
         and( xdot_b > V_bar0+eps_n1 , alpha_bar < pi/2 ) )
    decelerating = 1;
    switching_side = 1;
    % switch side flag state
    state = 4;     
% % move the UAV to the other side of the buoy to be able to decelerate:    
% elseif and( is_active == 0 && decelerating == 0 && switching_side == 0,...
%         not(and(abs(x_rel-x_rel_final) <= 0.05, alpha_bar > pi/2) ))
% %        not(and(abs(alpha-alpha_bar_step) <= 0.5*(pi/180), alpha_bar > pi/2) ))
%     is_active = 0;
%     decelerating = 1; 
%     switching_side = 1;
%     % switching side state
%     c = 7; 
% Stop switching side and prepare to return to elevation hold with (alpha > pi/2):    
elseif and( is_active == 0 && decelerating == 1 && switching_side == 1,...
         and(abs(x_rel-x_rel_final) <= dx_thr, alpha_bar > pi/2  ))
    % and(abs(alpha_bar_step-alpha_bar_switch) <= 1*(pi/180) ,...
    switching_side = 0;
    % switching side stop state
    state = 5;
% activate deceleration action (alpha > pi/2):    
elseif and( is_active == 0 && decelerating == 1 && switching_side == 0,...
         and(alpha_bar > pi/2 , xdot_b > V_bar0+eps_n1 )  )
    is_active = 1;
    % switching side stop state
    state = 6;  
% % Keep deceleration:    
% elseif and( is_active == 1 && decelerating == 1 && switching_side == 0,...
%         and(alpha_bar > pi/2 , xdot_b > V_bar0-eps_p1 )  )
%     is_active = 1;
%     decelerating = 1; 
%     switching_side = 0;    
%     c = 10;    
% stop decelerating after velocity error is reduced ...
% or if the system has decoupled (removed for testing):    
elseif and( is_active == 1 && decelerating == 1 && switching_side == 0,...
        and(alpha_bar > pi/2 , or( (xdot_b <= V_bar0-eps_p1), 0 ))) % (r < r_thr)
    is_active = 0;
    state = 7;
% % keep deactivated since velocity error has not reached the threshold:    
% elseif and( is_active==0  && decelerating==1 && switching_side==0 && alpha>pi/2,...
%         and( xdot_b < V_bar0+eps_n1 , xdot_b > V_bar0-eps_p2 ) ) 
%     is_active = 0;
%     decelerating = 1; 
%     switching_side = 0;
%     % backwark elevation-hold state
%     c = 12;     
% prepare to accelerate since velocity is too low:    
elseif and( is_active == 0  && decelerating == 1 && switching_side == 0,...
        and( xdot_b < V_bar0-eps_p2 , alpha > pi/2 ) ) 
    decelerating = 0; 
    % accelerate flag state
    state = 8;      
% declare UAV switching side state (to forward):    
elseif and( is_active == 0 && decelerating == 0 && switching_side == 0,...
         and( xdot_b < V_bar0-eps_p1 , alpha_bar > pi/2 ) )
     switching_side = 1;
    % switch side flag state
    state = 9;     
% % move the UAV to the other (front) side of the buoy to be able to decelerate:    
% elseif and( is_active == 0 && decelerating == 0 && switching_side == 1,...
%         not(and(abs(alpha-alpha_bar) <= 1*(pi/180), alpha_bar < pi/2) ))
%     is_active = 0;
%     decelerating = 0; 
%     switching_side = 1;
%     % switching side state
%     c = 15; 
% Stop switching side and prepare to return to elevation hold with (alpha < pi/2):    
elseif and( is_active == 0 && decelerating == 0 && switching_side == 1,...
         and(abs(x_rel-x_rel_final) <= dx_thr, alpha_bar < pi/2)  )    
    switching_side = 0;
    % switching side stop state
    state = 10;    
% need completion for other cases (to switch from backward to forward motion)...    
end    

    
%%
c           = state;
active      =  is_active;
decelerate  =  decelerating;   
switch_side =  switching_side;

== matlab function Marine_LocoMotive_UAV/Sensors and Filters/Data processing/Estimate Attitude/Calculate Roll and Pitch (From Acceleration Data)/calc_roll_pitch ==
  data: roll_acc output; pitch_acc output; acc_body input
function [roll_acc, pitch_acc]   = fcn(acc_body)
%#eml
n = norm(acc_body,2);
if n>eps
    acc_body = -acc_body/n; 
else
    acc_body = [0 0 1]';
end

roll_acc = atan2(acc_body(2),acc_body(3));
pitch_acc = atan2( -acc_body(1), acc_body(2)*sin(roll_acc)+acc_body(3)*cos(roll_acc));

== matlab function Marine_LocoMotive_UAV/Sensors and Filters/Data processing/Estimate Position/Kalman Filter - Height ==
  settings: updateMethod=DISCRETE  sampleTime=T
  data: height output; optitrack input; sonar_d input; dt input; x0 input
function height   = fcn(optitrack,sonar_d,dt,x0)
%#eml

     Q_sonar  = 0.1; %0.01; %0.001
     Q_optitrack   = 0.01; %0.01;  %0.003
     R_height =  0.03;  %0.03

    
    persistent P_00;
    persistent P_01;
    persistent P_10;
    persistent P_11;
    persistent x_height;
    persistent x_bias;
        
    if isempty(P_00)
        P_00 = 0;
    end
    
    if isempty(P_01)
        P_01 = 0;
    end
    if isempty(P_10)
        P_10 = 0;
    end
    if isempty(P_11)
        P_11 = 0;
    end
    if isempty(x_bias)
       x_bias = 0;
    end
    if isempty(x_height)
       x_height = x0;
    end
    
    
    % Compensate for sonar rate calculation (sonar sample rate is 10Hz)
    sonar_d_corrected = sonar_d*dt*10;  % m/s
    
    % Reject large height rate changes from sonar
    % As those are likely a result of obstacle underneath or noise
    if(abs(sonar_d_corrected) > 1 )    % max height rate (m/s)
        sonar_d_corrected = 0;
    end
    
    % Calculate the new output
    %x_height = x_height + dt * (sonar_d - x_bias); % old 
    x_height = x_height + dt * (sonar_d_corrected - x_bias);
    P_00 = P_00 -  dt * (P_10 + P_01) + Q_sonar * dt;
    P_01 = P_01  - dt * P_11;
    P_10 = P_10  - dt * P_11;
    P_11 = P_11  + Q_optitrack * dt;

    % Assuming H = [0.95 (effect of optitrack) 0.05 (effect of sonar)]
    e = (0.05*x_height + 0.95*optitrack) - x_height;
    S = P_00 + R_height;
    K_0 = P_00 / S;
    K_1 = P_10 / S;

    % Correction
    x_height = x_height+  K_0 * e;
    x_bias  = x_bias+  K_1 * e;
    P_00 = P_00 - K_0 * P_00;
    P_01 = P_01 - K_0 * P_01;
    P_10 = P_10 - K_1 * P_00;
    P_11 = P_11 - K_1 * P_01;

    height = x_height;
